simulink subsystem "limit_joint_coordinates_ref_subsys"  (R2022b)
settings: Solver=VariableStepAuto  StartTime=0.0  StopTime=10.0  RelTol=1e-3
undefined symbols (not defined in the file): param_robot, q_0
settings Model: Creator=emu  LastModifiedBy=emu

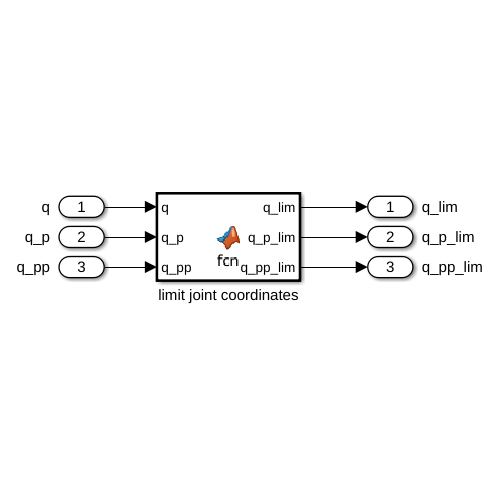
[thumbnail: Simulink's stored preview of the top-level diagram]
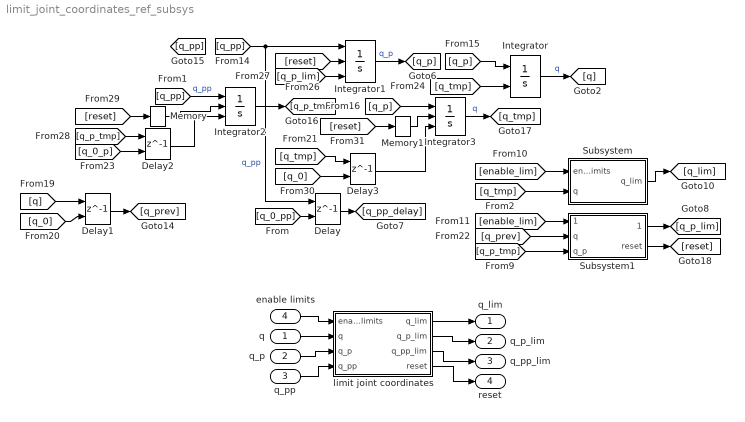
== system limit_joint_coordinates_ref_subsys ==
  q : Inport
  q_p : Inport  Port=2
  q_pp : Inport  Port=3
  enable limits : Inport  Port=4
  Delay{,1..3} (4 alike) : Delay  DelayLength=1  InitialConditionSource=Input port
      settings: InputPortMap=u0,p4
  Integrator : Integrator  InitialConditionSource=external  InitialCondition=q_0  UpperSaturationLimit=param_robot.q_limit_upper  LowerSaturationLimit=param_robot.q_limit_lower
  Integrator1 : Integrator  ExternalReset=level hold  InitialConditionSource=external  InitialCondition=param_robot.q_0_p_ref  UpperSaturationLimit=param_robot.q_p_limit_upper  LowerSaturationLimit=param_robot.q_p_limit_lower
  Integrator2 : Integrator  ExternalReset=level hold  InitialConditionSource=external  InitialCondition=param_robot.q_0_p_ref  UpperSaturationLimit=param_robot.q_p_limit_upper  LowerSaturationLimit=param_robot.q_p_limit_lower
  Integrator3 : Integrator  ExternalReset=level hold  InitialConditionSource=external  InitialCondition=q_0  UpperSaturationLimit=param_robot.q_limit_upper  LowerSaturationLimit=param_robot.q_limit_lower
  Memory : Memory
  Memory1 : Memory
  Subsystem : Subsystem
  Subsystem1 : Subsystem
  limit joint coordinates : MATLAB Function  TreatAsAtomicUnit=on
  q_lim : Outport
  q_p_lim : Outport  Port=2
  q_pp_lim : Outport  Port=3
  reset : Outport  Port=4
  wires:
  enable limits/1 -> limit joint coordinates/1(enable_limits)
  limit joint coordinates/4(reset) -> reset/1
  q_p/1 -> limit joint coordinates/3(q_p)
  q_pp/1 -> limit joint coordinates/4(q_pp)
  limit joint coordinates/3(q_pp_lim) -> q_pp_lim/1
  limit joint coordinates/2(q_p_lim) -> q_p_lim/1
  q/1 -> limit joint coordinates/2(q)
  limit joint coordinates/1(q_lim) -> q_lim/1
  [q_pp] -> Delay/1, Integrator1/1  "q_pp"
  [reset] -> Memory1/1
  Integrator/1 -> [q]  "q"
  [q_prev] -> Subsystem1/2(q)
  Delay2/1 -> Integrator2/3
  [q_p_tmp] -> Delay2/1
  [q_0_p] -> Delay2/2
  [q_0] -> Delay3/2
  Integrator3/1 -> [q_tmp]  "q"
  [q_p] -> Integrator3/1
  [q_tmp] -> Subsystem/2(q)
  [q_p] -> Integrator/1
  [q_0] -> Delay1/2
  [q_0_pp] -> Delay/2
  Delay/1 -> [q_pp_delay]
  Delay1/1 -> [q_prev]
  Integrator2/1 -> [q_p_tmp]
  [enable_lim] -> Subsystem1/1(enable limits)
  [q_tmp] -> Delay3/1
  [reset] -> Memory/1
  Subsystem1/1(q_pp_lim) -> [q_p_lim]
  Subsystem/1(q_lim) -> [q_lim]
  ? -> [q_pp]  "q_pp"
  [enable_lim] -> Subsystem/1(enable limits)
  [q_pp] -> Integrator2/1  "q_pp"
  [q_p_tmp] -> Subsystem1/3(q_p)
  [q_p_lim] -> Integrator1/3
  [q] -> Delay1/1
  Delay3/1 -> Integrator3/3
  Subsystem1/2(reset) -> [reset]
  Integrator1/1 -> [q_p]  "q_p"
  [reset] -> Integrator1/2
  Memory/1 -> Integrator2/2
  Memory1/1 -> Integrator3/2
  [q_tmp] -> Integrator/2

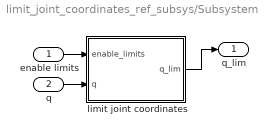
== system limit_joint_coordinates_ref_subsys/Subsystem ==
  enable limits : Inport
  q : Inport  Port=2
  limit joint coordinates : MATLAB Function  TreatAsAtomicUnit=on
  q_lim : Outport
  wires:
  q/1 -> limit joint coordinates/2(q)
  enable limits/1 -> limit joint coordinates/1(enable_limits)
  limit joint coordinates/1(q_lim) -> q_lim/1

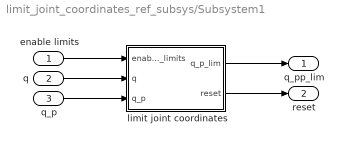
== system limit_joint_coordinates_ref_subsys/Subsystem1 ==
  enable limits : Inport
  q : Inport  Port=2
  q_p : Inport  Port=3
  limit joint coordinates : MATLAB Function  TreatAsAtomicUnit=on
  q_pp_lim : Outport
  reset : Outport  Port=2
  wires:
  limit joint coordinates/2(reset) -> reset/1
  q/1 -> limit joint coordinates/2(q)
  q_p/1 -> limit joint coordinates/3(q_p)
  limit joint coordinates/1(q_p_lim) -> q_pp_lim/1
  enable limits/1 -> limit joint coordinates/1(enable_limits)

== matlab function limit_joint_coordinates_ref_subsys/limit joint coordinates ==
  data: enable_limits input; q input; q_lim output; q_p input; q_pp input; q_p_lim output; q_pp_lim output; param_robot parameter; reset output
function [q_lim, q_p_lim, q_pp_lim, reset] = fcn(enable_limits, q, q_p, q_pp, param_robot)

if(enable_limits == 1)
    q_lim = min(max(q, param_robot.q_limit_lower), param_robot.q_limit_upper);
    q_p_lim = min(max(q_p, param_robot.q_p_limit_lower), param_robot.q_p_limit_upper);
    q_pp_lim = min(max(q_pp, param_robot.q_pp_limit_lower), param_robot.q_pp_limit_upper);
    
    n = param_robot.n_DOF;
    
    % naja wenn gelenk in den grenzen sind kann die geschw. in die eine
    % richtung nur 0 sein.. -> sonst vertut man sich bein integrieren
    Q_ub = 1/2 * eye(n) - 1/4 * (1 + my_sign(q_p)) * diag(my_sign(q - param_robot.q_limit_upper));
    Q_lb = 1/2 * eye(n) + 1/2 * (1 - my_sign(q_p)) * diag(my_sign(q - param_robot.q_limit_lower));
    Q_lim = Q_ub * Q_lb;
    
    % wenn man in den limits is kann klarerweise keine geschw. in den
    % joints vorliegen, aber das führt zu sprüngen in C(q,qp)qp
    %q_p_lim = Q_lim * q_p_lim;
    %q_pp_lim = Q_lim * q_pp_lim;
    
    if(sum(Q_lim, 'all') < n)
        reset=1;
    else
        reset=0;
    end
else
    q_lim = q;
    q_p_lim = q_p;
    q_pp_lim = q_pp;
    reset = 0;
end

end

function my_sign = my_sign(x)
    my_sign = 2*(x >= 0) - 1;
end

== matlab function limit_joint_coordinates_ref_subsys/Subsystem/limit joint coordinates ==
  data: enable_limits input; q input; q_lim output; param_robot parameter
function q_lim  = fcn(enable_limits, q, param_robot)

if(enable_limits == 1)
    q_lim = min(max(q, param_robot.q_limit_lower), param_robot.q_limit_upper);

else
    q_lim = q;
end

end

== matlab function limit_joint_coordinates_ref_subsys/Subsystem1/limit joint coordinates ==
  data: enable_limits input; q input; q_p input; q_p_lim output; param_robot parameter; reset output
function [q_p_lim,reset] = fcn(enable_limits, q, q_p, param_robot)

if(enable_limits == 1)
    q_p_lim = min(max(q_p, param_robot.q_p_limit_lower), param_robot.q_p_limit_upper);
    
    n = param_robot.n_DOF;
    
    % naja wenn gelenk in den grenzen sind kann die geschw. in die eine
    % richtung nur 0 sein.. -> sonst vertut man sich bein integrieren
    Q_ub = 1/2 * eye(n) - 1/2 * diag(my_sign(q - param_robot.q_limit_upper));
    Q_lb = 1/2 * eye(n) + 1/2 * diag(my_sign(q - param_robot.q_limit_lower));
    Q_lim = Q_ub * Q_lb;
    
    % wenn man in den limits is kann klarerweise keine geschw. in den
    % joints vorliegen, aber das führt zu sprüngen in C(q,qp)qp
    q_p_lim = Q_lim * q_p_lim;
    if(sum(Q_lim, 'all') < n)
        reset=1;
    else
        reset=0;
    end
else
    q_p_lim = q_p;
    reset=0;
end

end

function my_sign = my_sign(x)
    my_sign = 2*(x > 0) - 1;
end
